simulink model "sensorFusionWithControlBackup"  (R2024a)
settings: Solver=FixedStepAuto  StartTime=0.0  StopTime=inf  FixedStep=controlRate  RelTol=1e-3  EnableMultiTasking=on
values from neighbouring files (symbols this model uses):
  A_pend = [0 1 0 0 ... (first row only)    [initModelMatrices.m]
  B_pend = [0; (m^2*l^2*g)/p*1/(m+M); 0; -(m*l)/p]    [initModelMatrices.m]
undefined symbols (not defined in the file or in its folder): accelToUnit, Ad_aug, angleEstRate, Bd_aug, Cd_aug, controlRate, CPR, D_min, DiscIntNeverNeededParam, Discrete, Dmin, gyroToUnit, K_aug_lqr, K_lqr, MaxMotorVoltage, Q_ang_kf, Q_aug_kf, Q_kf, R_ang_kf, R_aug_kf, R_kf, stateEstRate, Time, wheelBase, wheelRadius
libraries: stm32f4xxblockslib x13, dspstat3 x6, stm32blockslib x2, stm32f7xxblockslib x2, slpidlib x1, ctrlSharedLib x1
(part 2 of 2)

== matlab function sensorFusionWithControlBackup/Kalman 2D/KalmanFilter/MATLAB Function ==
  data: ax input single; tiltAngle output single; ay input single; az input single; gx input single; gy input single; sampleTime input single; Q_kf input single; R_kf input single; measRollPitch output single
function [tiltAngle,measRollPitch] = kalman2D(ax, ay, az, gx, gy,sampleTime,Q_kf,R_kf)
%#codegen

persistent x P instance

dt = single(sampleTime); % Sample time
deg2rad = single(pi / 180);

% Initialize persistent state vector and covariance matrix
if isempty(instance)
    % State: [theta_x; theta_y; omega_x; omega_y]
    x = single(zeros(4, 1));
    P = single(eye(4) * 0.1);
    instance = true;
end

% System dynamics matrix
A = single([1 0 dt 0;
             0 1 0 dt;
             0 0 1  0;
             0 0 0  1]);

% Process noise covariance (tune as needed)
Q = single(Q_kf);

% Measurement matrix: we only measure [theta_x, theta_y]
H = single([1 0 0 0;
            0 1 0 0]);

% Measurement noise covariance
R = single(R_kf);

% ====== PREDICT STEP ======

% Inject new gyro measurements into angular rate state (rad/s)!!!!!!!!!!!!
x(3) = gy * deg2rad;
x(4) = gx * deg2rad;

% Can be:
   % B = single([0 0;
   %              0 0;
   %              1 0;
   %              0 1]);
   % 
   %  % ===== PREDICT STEP =====
   %  % Gyro control input (rad/s)
   %  u = [gx; gy] * deg2rad;
   % 
   %  % Predict next state
   %  x = A * x + B * u;

% Predict state and covariance
x = A * x;
P = A * P * A' + Q;

% ====== MEASUREMENT FROM ACCELEROMETER ======

% Estimate roll and pitch from accelerometer
roll_meas  = atan2(ax,az);
% pitch_meas = atan(-ax / sqrt(ay^2 + az^2));
pitch_meas = atan2(ay,az);
z = [roll_meas; pitch_meas];

measRollPitch = z;


% ====== UPDATE STEP ======
K = P * H' / (H * P * H' + R);
x = x + K * (z - H * x);
P = (eye(4) - K * H) * P;

% Output estimated [roll; pitch]
tiltAngle = x(1:2);
end

== matlab function sensorFusionWithControlBackup/Robot state estimation Kalman filter/Main Kalman filter/Main Kalman 1D/MATLAB Function ==
  data: tiltAngle input single; x_hat_states output single; x_pos input single; y_pos input single; u input; A_pend input; B_pend input; Q_pend input; R_pend input
function x_hat_states = mainKalman(tiltAngle,x_pos,y_pos,u, A_pend, B_pend, Q_pend, R_pend)
% kalman_filter  Discrete-time Kalman filter for 2-wheeled self-balancing robot
% States: x = [ x; x_dot; theta; theta_dot ]  (4x1)
% Measurements assumed y = [ x_encoder; theta_accel; theta_dot_gyro ] (3x1)
%
% Inputs:
%   y   (3x1)   measurement vector
%   u   (1x1)   control input
%   A   (4x4)   state transition matrix (discrete)
%   B   (4x1)   input matrix
%   Q   (4x4)   process noise covariance
%   R   (3x3)   measurement noise covariance
%   x0  (4x1)   initial state (used on reset)
%   P0  (4x4)   initial covariance (used on reset)
%   reset (scalar logical/int)  set to 1 to reinitialize x_hat := x0, P := P0
%
% Outputs:
%   x_hat (4x1)  filtered state estimate
%   P_out (4x4)  current covariance
%
% NOTE: This code uses single precision to be suitable for embedded targets.

    A = single(A_pend);
    B = single(B_pend);
    Q = single(Q_pend);
    R = single(R_pend);
    y = single([tiltAngle;x_pos]);

    % Voltage to force conversion in motor steady state
    params.N = 42;
    params.Kt = 0.005671;
    params.eta = 0.9;
    params.Ke = 0.3; 
    params.R = 3.428571;
    params.useBackEmf = false;
    params.r = 0.03;
    F = V_to_force(u, 0, params);

    u = single(F);
    
    % Dimensions (hard-coded to avoid dynamic size issues)
    nx = 4;   % state dimension
    nz = 2;   % measurement dimension (y size)
    
    persistent xhat P initialized

    if isempty(initialized)
        xhat = zeros(nx,1,'single');
        P    = eye(nx,'single') * single(1e-3);
        initialized = true;
    end
    
        H = single([ 1 0 0 0;    % x_encoder measures x
                     0 0 1 0]);   % theta
        
        % Prediction step
        x_pred = A * xhat + B * u;           % 4x1
        P_pred = A * P * A' + Q;             % 4x4
        
        % Update step
        y_pred = H * x_pred;                  % 2x1
        innov = y - y_pred;                   % 2x1
        
        % Innovation covariance S = H*P_pred*H' + R  (2x2)
        S = H * P_pred * H' + R;
        
        % Kalman gain K = P_pred * H' * inv(S)  (4x2)
        S_inv = inv(S);                       % 2x2
        K = P_pred * H' * S_inv;              % 4x2
        
        % State update
        xhat = x_pred + K * innov;            % 4x1
        
        % Joseph stabilized covariance update:
        I = eye(nx,'single');
        P = (I - K*H) * P_pred * (I - K*H)' + K * R * K';
        
        % Outputs
        x_hat_states = xhat;
        %P_out = P;
    
end

function F = V_to_force(V, omega_w, params)
% V_to_force  Convert applied voltage (V) to wheel force (N) - steady-state approx
%   V         : applied motor voltage (scalar) [V]
%   omega_w   : wheel angular speed (rad/s) (scalar)
%   params    : struct with fields
%       R    - motor resistance (ohm)
%       Kt   - torque constant (N*m/A)
%       Ke   - back-emf constant (V/(rad/s))
%       N    - gearbox ratio (omega_motor / omega_wheel)
%       r    - wheel radius (m)
%       eta  - drivetrain efficiency (0..1) (default 1)
%       useBackEmf - boolean (default true)
%
% Output:
%   F : force at wheel (N)

if ~isfield(params,'eta'), params.eta = 1; end
if ~isfield(params,'useBackEmf'), params.useBackEmf = true; end

R  = params.R;
Kt = params.Kt;
Ke = params.Ke;
N  = params.N;
r  = params.r;
eta = params.eta;

% linear gain (N/V)
alpha = (eta * N * Kt) / (r * R);

if params.useBackEmf
    % back-emf term (depends on wheel speed)
    beta = - (eta * N^2 * Kt * Ke) / (r * R);
    F = alpha * V + beta * omega_w;
else
    F = alpha * V;
end

end

== matlab function sensorFusionWithControlBackup/Subsystem1/MATLAB Function2 ==
  data: x output single; x_h input uint8; x_l input uint8; y_h input uint8; y_l input uint8; z_h input uint8; z_l input uint8; y output single; z output single; phyUnit input single
function [x, y, z] = convert_raw_units(x_h, x_l, y_h, y_l, z_h, z_l, phyUnit)

    % Combine LSB and MSB (signed 16-bit)
    x_raw = typecast(bitor(bitshift(uint16(x_h),8), uint16(x_l)), 'int16');
    y_raw = typecast(bitor(bitshift(uint16(y_h),8), uint16(y_l)), 'int16');
    z_raw = typecast(bitor(bitshift(uint16(z_h),8), uint16(z_l)), 'int16');
    
    % Convert to physical units
    % ITG3200: 14.375 LSBs per °/sec
    x = single(x_raw) / phyUnit;
    y = single(y_raw) / phyUnit;
    z = single(z_raw) / phyUnit;
    
end
